simulink model "simulink_problem12"  (R2019b)
settings: Solver=VariableStepAuto  StartTime=0.0  StopTime=2  RelTol=1e-3
values from neighbouring files (symbols this model uses):
  d1 = [J_eff(1)  (f_eff + KT*KD1)  KT*KP1]    [problem12.m]    (also in problem15.m = [J_eff(1)  (f_eff + KT*KD1)  KT*KP1  KT*KI]; problem16.m = [J_eff(1)  (f_eff + KT*KD1)  KT*KP1  KT*KI]; problem17.m = 1.5; problem18.m = 1.5)
  d2 = [J_eff(2)  (f_eff + KT*KD2)  KT*KP2]    [problem12.m]    (also in problem15.m = [J_eff(2)  (f_eff + KT*KD2)  KT*KP2  KT*KI]; problem16.m = [J_eff(2)  (f_eff + KT*KD2)  KT*KP2  KT*KI])
  d3 = [J_eff(3)  (f_eff + KT*KD3)  KT*KP3]    [problem12.m]    (also in problem15.m = [J_eff(3)  (f_eff + KT*KD3)  KT*KP3  KT*KI]; problem16.m = [J_eff(3)  (f_eff + KT*KD3)  KT*KP3  KT*KI])
  d4 = [J_eff(4)  (f_eff + KT*KD4)  KT*KP4]    [problem12.m]    (also in problem15.m = [J_eff(4)  (f_eff + KT*KD4)  KT*KP4  KT*KI]; problem16.m = [J_eff(4)  (f_eff + KT*KD4)  KT*KP4  KT*KI])
  n1 = KT * [KD1  KP1]    [problem12.m]    (also in problem15.m = KT * [KD1  KP1  KI]; problem16.m = KT * [KD1  KP1  KI])
  n2 = KT * [KD2  KP2]    [problem12.m]    (also in problem15.m = KT * [KD2  KP2  KI]; problem16.m = KT * [KD2  KP2  KI])
  n3 = KT * [KD3  KP3]    [problem12.m]    (also in problem15.m = KT * [KD3  KP3  KI]; problem16.m = KT * [KD3  KP3  KI])
  n4 = KT * [KD4  KP4]    [problem12.m]    (also in problem15.m = KT * [KD4  KP4  KI]; problem16.m = KT * [KD4  KP4  KI])
settings Model: Creator=ben  LastModifiedBy=axeljacobsen

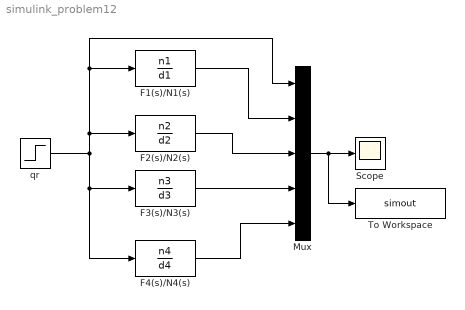
== system simulink_problem12 ==
  F1(s)/N1(s) : TransferFcn  Numerator=n1  Denominator=d1
  F2(s)/N2(s) : TransferFcn  Numerator=n2  Denominator=d2
  F3(s)/N3(s) : TransferFcn  Numerator=n3  Denominator=d3
  F4(s)/N4(s) : TransferFcn  Numerator=n4  Denominator=d4
  Mux : Mux  Inputs=5
  Scope : Scope
  To Workspace : ToWorkspace  VariableName=simout  SampleTime=-1
  qr : Step  Time=0.5  After=0.34  SampleTime=0
  wires:
  qr/1 -> F2(s)/N2(s)/1, F1(s)/N1(s)/1, Mux/1, F4(s)/N4(s)/1, F3(s)/N3(s)/1
  F1(s)/N1(s)/1 -> Mux/2
  F2(s)/N2(s)/1 -> Mux/3
  F3(s)/N3(s)/1 -> Mux/4
  F4(s)/N4(s)/1 -> Mux/5
  Mux/1 -> To Workspace/1, Scope/1
